simulink model "MyDrivelIne"  (R2018b)
settings: Solver=VariableStepAuto  StartTime=0.0  StopTime=10.0  RelTol=1e-3
libraries: autolibsharedcoupling x3, autolibutils x1, vehdynlibsteering x1, autolibshareddiff x1, autolibsharedtransfixedgear x1
settings Model: Creator=ivory  LastModifiedBy=ivory

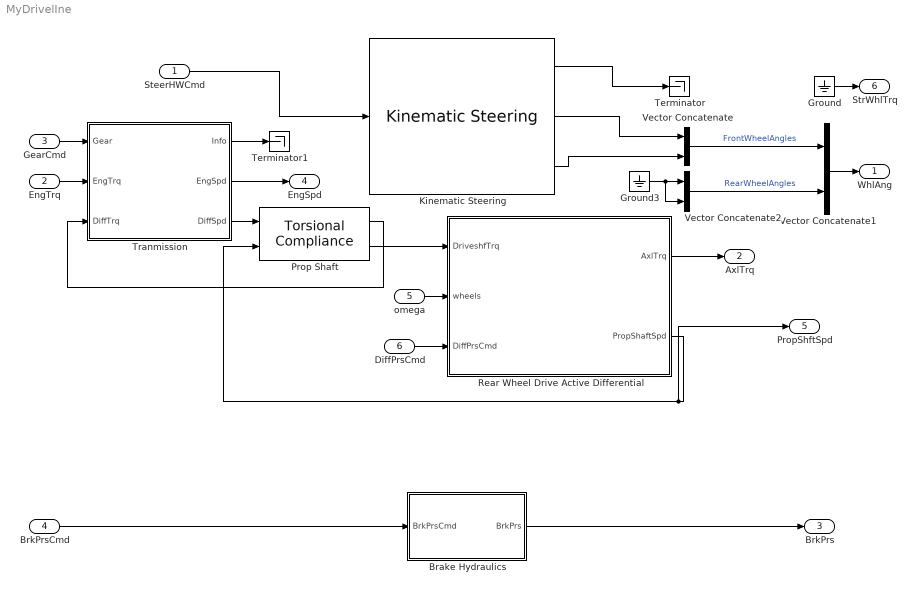
== system MyDrivelIne ==
  SteerHWCmd : Inport
  EngTrq : Inport  Port=2
  GearCmd : Inport  Port=3
  BrkPrsCmd : Inport  Port=4  PortDimensions=4
  omega : Inport  Port=5
  DiffPrsCmd : Inport  Port=6
  Brake Hydraulics : Subsystem
  Ground : Ground
  Ground3 : Ground
  Kinematic Steering : vehdynlibsteering/Kinematic Steering  StrgType=Ackerman  StrgRatioType=Constant  Loc=Front  NrmlFctr=1  TrckWdth=1.922  WhlBase=(1.515+1.504)  Db=0  StrgRng=3*pi  StrgAngBpts="[-6.2832   -5.0265   -3.7699   -2.5133   -1.2566         0    1.2566    2.5133    3.7699    5.0265    6.2832]"  StrgRatioTbl=|  StrgRatio=18  StrgArmLngth=0.1  RckCsLngth=0.5  TieRodLngth=0.248  D=0.2  PnnRadius=0.0057  PnnRadiusTbl="[0.0055    0.0055    0.0056    0.0057    0.0058    0.0057    0.0057    0.0057    0.0056    0.0055    0.0055]"  RodLngth=0.1  ParaArmLngth=0.9  aMode=2
      | [13.5000   13.3750   13.2500   13.1250   13.0000   13.0000   13.0000   13.1250   13.2500   13.3750   13.5000
      | ]
      settings: SourceProductName=Vehicle Dynamics Blockset
  Prop Shaft : autolibsharedcoupling/Torsional Compliance  port_config=Simulink  k=5e3  b=100  theta_o=0  domega_o=0  omega_c=150  blkID=0  aMode=2
      settings: SourceProductName=Powertrain Blockset  SourceProductBaseCode=PW
  Rear Wheel Drive Active Differential : Subsystem
  Terminator : Terminator
  Terminator1 : Terminator
  Tranmission : Subsystem
  Vector Concatenate : Concatenate
  Vector Concatenate1 : Concatenate
  Vector Concatenate2 : Concatenate
  WhlAng : Outport  Unit=rad
  AxlTrq : Outport  Port=2
  BrkPrs : Outport  Port=3  PortDimensions=4
  EngSpd : Outport  Port=4
  PropShftSpd : Outport  Port=5
  StrWhlTrq : Outport  Port=6  Unit=N*m
  wires:
  Ground3/1 -> Vector Concatenate2/2, Vector Concatenate2/1
  Kinematic Steering/1 -> Terminator/1
  Kinematic Steering/3 -> Vector Concatenate/2
  Vector Concatenate1/1 -> WhlAng/1
  Vector Concatenate2/1 -> Vector Concatenate1/2  "RearWheelAngles"
  Vector Concatenate/1 -> Vector Concatenate1/1  "FrontWheelAngles"
  Kinematic Steering/2 -> Vector Concatenate/1
  Ground/1 -> StrWhlTrq/1
  Rear Wheel Drive Active Differential/1(AxlTrq) -> AxlTrq/1
  BrkPrsCmd/1 -> Brake Hydraulics/1(BrkPrsCmd)
  Brake Hydraulics/1(BrkPrs) -> BrkPrs/1
  Tranmission/1(Info) -> Terminator1/1
  Tranmission/2(EngSpd) -> EngSpd/1
  Tranmission/3(DiffSpd) -> Prop Shaft/1
  Prop Shaft/1 -> Tranmission/3(DiffTrq)
  Prop Shaft/2 -> Rear Wheel Drive Active Differential/1(DriveshfTrq)
  omega/1 -> Rear Wheel Drive Active Differential/2(wheels)
  DiffPrsCmd/1 -> Rear Wheel Drive Active Differential/3(DiffPrsCmd)
  Rear Wheel Drive Active Differential/2(PropShaftSpd) -> PropShftSpd/1, Prop Shaft/2
  SteerHWCmd/1 -> Kinematic Steering/1
  EngTrq/1 -> Tranmission/2(EngTrq)
  GearCmd/1 -> Tranmission/1(Gear)

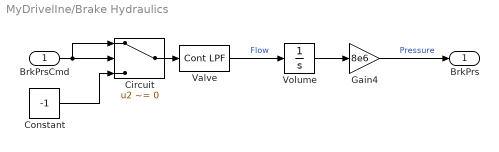
== system MyDrivelIne/Brake Hydraulics ==
  BrkPrsCmd : Inport
  Circuit : Switch  Criteria=u2 ~= 0
  Constant : Constant  Value=-1
  Gain4 : Gain  Gain=8e6
  Valve : autolibutils/Cont LPF  wc=200*2*pi  aMode=2
      settings: SourceProductName=Powertrain Blockset  SourceProductBaseCode=PW
  Volume : Integrator  LimitOutput=on  UpperSaturationLimit=1  LowerSaturationLimit=0  AbsoluteTolerance=1e-3
  BrkPrs : Outport
  wires:
  Volume/1 -> Gain4/1
  Valve/1 -> Volume/1  "Flow"
  BrkPrsCmd/1 -> Circuit/1, Circuit/2
  Gain4/1 -> BrkPrs/1  "Pressure"
  Circuit/1 -> Valve/1
  Constant/1 -> Circuit/3

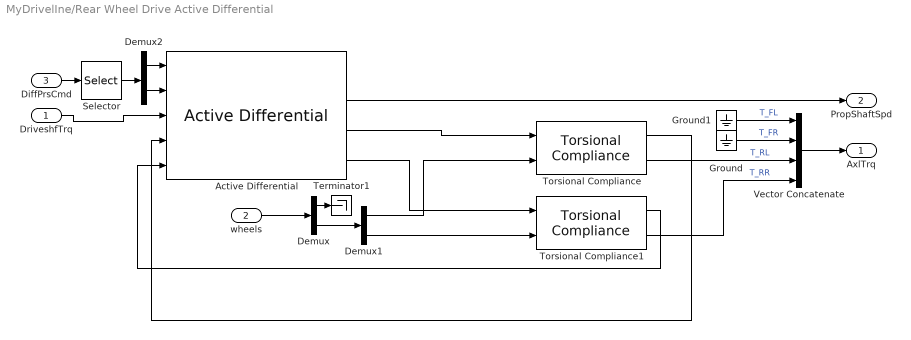
== system MyDrivelIne/Rear Wheel Drive Active Differential ==
  DriveshfTrq : Inport
  wheels : Inport  Port=2
  DiffPrsCmd : Inport  Port=3
  Active Differential : autolibshareddiff/Active Differential  diffType=Spur gears, superposition clutches  Ns1=.875  Ns2=1.125  Jgc=.003  Np1=1.125  Js1=.001  Jc1=.001  Jr1=.002  Np2=1.125  Js2=.001  Jc2=0.001  Jr2=0.002  shaftSwitchMask=To the left of center-line  Ndiff=4  Jd=.1  bd=1e-3  Jw1=.1  bw1=1e-3  Jw2=.1  bw2=1e-3  omegaw1o=0  omegaw2o=0  couplingType=Pre-loaded ideal clutch  Aeff=0.01  Ndisks=4  Reff=.20  Fc=500  muc=[.16 0.13 0.115 0.11 0.105 0.1025 0.10125 .10125]  dw=[0 10 20 40 60 80 100 500]  TdPdw=[-1000, -500, -90, -50, -5, 0, 5, 50, 90, 500, 1000].*ones(11)  pT=[0 1e3 5e3 7e3 1e4 2e4 5e4 1e5 5e5 1e6 5e6]  dwT=[-500 -200, -175, -100, - 50, 0, 50, 100, 175, 200, 500]  tauC=.01  IdealInterpMethod=Linear point-slope  IdealExtrapMethod=Clip  TdwInterpMethod=Linear point-slope  TdwExtrapMethod=Clip  maxAbsSpd=5e3  aMode=2  blkID=0
      settings: SourceProductName=Powertrain Blockset  SourceProductBaseCode=PW
  Demux : Demux  Outputs=[2,2]
  Demux1 : Demux  Outputs=2
  Demux2 : Demux  Outputs=2
  Ground : Ground
  Ground1 : Ground
  Selector : Selector  InputPortWidth=4  IndexOptions=Index vector (dialog)  Indices=[3 4]  OutputSizes=1
  Terminator1 : Terminator
  Torsional Compliance : autolibsharedcoupling/Torsional Compliance  port_config=Simulink  k=5e3  b=50  theta_o=0  domega_o=0  omega_c=150  blkID=0  aMode=2
      settings: SourceProductName=Powertrain Blockset  SourceProductBaseCode=PW
  Torsional Compliance1 : autolibsharedcoupling/Torsional Compliance  port_config=Simulink  k=5e3  b=50  theta_o=0  domega_o=0  omega_c=150  blkID=0  aMode=2
      settings: SourceProductName=Powertrain Blockset  SourceProductBaseCode=PW
  Vector Concatenate : Concatenate  NumInputs=4
  AxlTrq : Outport
  PropShaftSpd : Outport  Port=2
  wires:
  Selector/1 -> Demux2/1
  Ground/1 -> Vector Concatenate/2  "T_FR"
  Ground1/1 -> Vector Concatenate/1  "T_FL"
  Demux1/1 -> Torsional Compliance/2
  Vector Concatenate/1 -> AxlTrq/1
  Demux/1 -> Terminator1/1
  wheels/1 -> Demux/1
  Torsional Compliance1/2 -> Vector Concatenate/4  "T_RR"
  Torsional Compliance/2 -> Vector Concatenate/3  "T_RL"
  Active Differential/2 -> PropShaftSpd/1
  Active Differential/3 -> Torsional Compliance/1
  DiffPrsCmd/1 -> Selector/1
  DriveshfTrq/1 -> Active Differential/3
  Demux2/1 -> Active Differential/1
  Demux2/2 -> Active Differential/2
  Demux/2 -> Demux1/1
  Torsional Compliance/1 -> Active Differential/4
  Torsional Compliance1/1 -> Active Differential/5
  Demux1/2 -> Torsional Compliance1/2
  Active Differential/4 -> Torsional Compliance1/1

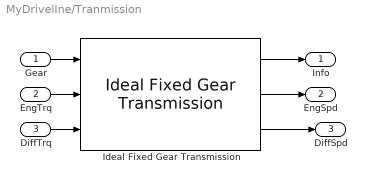
== system MyDrivelIne/Tranmission ==
  Gear : Inport
  EngTrq : Inport  Port=2
  DiffTrq : Inport  Port=3
  Ideal Fixed Gear Transmission : autolibsharedtransfixedgear/Ideal Fixed Gear Transmission  VariantControl=0  TransEffModelPopup=Gear only  gearInterp=Nearest  G=[-1,0,1,2,3,4,5,6,7,8]  Trq_bpts=[25, 50, 75, 100, 150, 200, 250]  omega_bpts=[52.4 78.5 105 131 157 183 209 262 314 419 524]  Temp_bpts=[313 358]  N=[-3.820000000000000,4.560000000000000,4.560000000000000,2.970000000000000,2.080000000000000,1.690000000000000,1.270000000000000,1,0.850000000000000,0.650000000000000]  Jout=[0.128000000000000,0.128000000000000,0.128000000000000,0.100000000000000,0.062000000000000,0.028000000000000,0.010000000000000,0.010000000000000,0.010000000000000,0.010000000000000]  bout=[0.003000000000000,1.000000000000000e-03,0.003000000000000,0.002500000000000,0.002000000000000,1.000000000000000e-03,1.000000000000000e-03,1.000000000000000e-03,1.000000000000000e-03,1.000000000000000e-03]  eta=[0.900000000000000,0.900000000000000,0.900000000000000,0.900000000000000,0.900000000000000,0.950000000000000,0.950000000000000,0.950000000000000,0.950000000000000,0.950000000000000]  eta_tbl=reshape([0.53 0.71 0.77 0.79 0.82 0.82 0.82 0.5 0.7 0.77 0.79 0.82 0.82 0.82 0.54 0.72 0.78 0.81 0.83 0.82 0.82 0.56 0.73 0.79 0.81 0.84 0.82 0.82 0.58 0.74 0.79 0.82 0.84 0.82 0.82 0.57 0.74 0.79 0.82 0.84 0.82 0.82 0.58 0.74 0.79 0.82 0.84 0.82 0.82 0.58 0.74 0.79 0.82 0.84 0.82 0.82 0.57 0.74 0.8 0.82 0.85 0.82 0.82 0.55 0.73 0.78 0.81 0.84 0.82 0.82 0.51 0.71 0.77 0.81 0.84 0.82 0.82 0.53 0.71 0.77 0.79 0.82 0.82 0.82 0.5 0.7 0.77 0.79 0.82 0.82 0.82 0.54 0.72 0.78 0.81 0.83 0.82 0.82 0.56 0.73 0.79 0.81 0.84 0.82 0.82 0.58 0.74 0.79 0.82 0.84 0.82 0.82 0.57 0.74 0.79 0.82 0.84 0.82 0.82 0.58 0.74 0.79 0.82 0.84 0.82 0.82 0.58 0.74 0.79 0.82 0.84 0.82 0.82 0.57 0.74 0.8 0.82 0.85 0.82 0.82 0.55 0.73 0.78 0.81 0.84 0.82 0.82 0.51 0.71 0.77 0.81 0.84 0.82 0.82 0.53 0.71 0.77 0.79 0.82 0.82 0.82 0.5 0.7 0.77 0.79 0.82 0.82 0.82 0.54 0.72 0.78 0.81 0.83 0.82 0.82 0.56 0.73 0.79 0.81 0.84 0.82 0.82 0.58 0.74 0.79 0.82 0.84 0.82 0.82 0.57 0.74 0.79 0.82 0.84 0.82 0.82 0.58 0.74 0.79 0.82 0.84 0.82 0.82 0.58 0.74 0.79 0.82 0.84 0.82 0.82 0.57 0.74 0.8 0.82 0.85 0.82 0.82 0.55 0.73 0.78 0.81 0.84 0.82 0.82 0.51 0.71 0.77 0.81 0.84 0.82 0.82 0.7 0.79 0.82 0.83 0.84 0.84 0.84 0.63 0.76 0.8 0.82 0.83 0.84 0.84 0.58 0.74 0.79 0.81 0.83 0.84 0.84 0.58 0.74 0.79 0.81 0.83 0.84 0.84 0.58 0.74 0.79 0.81 0.84 0.84 0.84 0.57 0.73 0.78 0.81 0.84 0.85 0.84 0.57 0.73 0.79 0.81 0.84 0.85 0.84 0.56 0.73 0.78 0.81 0.83 0.85 0.84 0.55 0.73 0.78 0.81 0.84 0.85 0.84 0.52 0.71 0.77 0.8 0.83 0.85 0.84 0.48 0.69 0.76 0.79 0.83 0.84 0.84 0.64 0.76 0.8 0.81 0.83 0.84 0.84 0.56 0.73 0.78 0.8 0.83 0.84 0.84 0.54 0.71 0.77 0.8 0.82 0.84 0.84 0.53 0.71 0.77 0.8 0.83 0.84 0.84 0.51 0.71 0.77 0.8 0.83 0.84 0.85 0.52 0.7 0.77 0.8 0.83 0.84 0.85 0.51 0.71 0.76 0.79 0.83 0.84 0.85 0.5 0.69 0.76 0.79 0.82 0.84 0.85 0.45 0.68 0.75 0.78 0.82 0.84 0.85 0.43 0.67 0.74 0.78 0.81 0.83 0.84 0.38 0.63 0.71 0.75 0.8 0.82 0.83 0.65 0.79 0.84 0.85 0.88 0.89 0.89 0.56 0.75 0.81 0.83 0.86 0.88 0.89 0.52 0.72 0.79 0.83 0.86 0.88 0.88 0.51 0.72 0.79 0.83 0.86 0.88 0.89 0.49 0.71 0.78 0.82 0.86 0.88 0.89 0.47 0.7 0.78 0.82 0.86 0.87 0.88 0.45 0.69 0.77 0.81 0.85 0.87 0.88 0.4 0.67 0.75 0.8 0.84 0.86 0.88 0.3 0.64 0.73 0.78 0.83 0.86 0.87 0.17 0.55 0.67 0.73 0.8 0.83 0.85 0.089 0.45 0.61 0.69 0.77 0.81 0.83 0.61 0.75 0.82 0.84 0.87 0.87 0.88 0.54 0.73 0.8 0.82 0.86 0.87 0.88 0.51 0.71 0.79 0.82 0.86 0.87 0.88 0.52 0.72 0.79 0.82 0.86 0.87 0.89 0.52 0.72 0.8 0.83 0.86 0.88 0.89 0.53 0.72 0.79 0.82 0.86 0.87 0.89 0.5 0.7 0.78 0.82 0.86 0.88 0.88 0.46 0.69 0.77 0.81 0.85 0.87 0.88 0.4 0.67 0.75 0.8 0.83 0.86 0.88 0.33 0.64 0.73 0.78 0.83 0.85 0.87 0.33 0.64 0.73 0.78 0.83 0.85 0.87 0.78 0.85 0.87 0.88 0.89 0.89 0.89 0.73 0.83 0.86 0.88 0.89 0.89 0.89 0.72 0.83 0.86 0.88 0.89 0.89 0.89 0.72 0.83 0.87 0.89 0.9 0.89 0.89 0.72 0.83 0.87 0.88 0.9 0.89 0.89 0.71 0.83 0.87 0.88 0.9 0.89 0.89 0.71 0.83 0.86 0.88 0.9 0.89 0.89 0.7 0.82 0.86 0.88 0.9 0.89 0.89 0.69 0.82 0.86 0.88 0.9 0.89 0.89 0.67 0.81 0.86 0.88 0.9 0.89 0.89 0.63 0.79 0.85 0.87 0.89 0.89 0.89 0.78 0.85 0.87 0.88 0.89 0.89 0.89 0.73 0.83 0.86 0.88 0.89 0.89 0.89 0.72 0.83 0.86 0.88 0.89 0.89 0.89 0.72 0.83 0.87 0.89 0.9 0.89 0.89 0.72 0.83 0.87 0.88 0.9 0.89 0.89 0.71 0.83 0.87 0.88 0.9 0.89 0.89 0.71 0.83 0.86 0.88 0.9 0.89 0.89 0.7 0.82 0.86 0.88 0.9 0.89 0.89 0.69 0.82 0.86 0.88 0.9 0.89 0.89 0.67 0.81 0.86 0.88 0.9 0.89 0.89 0.63 0.79 0.85 0.87 0.89 0.89 0.89 0.78 0.85 0.87 0.88 0.89 0.89 0.89 0.73 0.83 0.86 0.88 0.89 0.89 0.89 0.72 0.83 0.86 0.88 0.89 0.89 0.89 0.72 0.83 0.87 0.89 0.9 0.89 0.89 0.72 0.83 0.87 0.88 0.9 0.89 0.89 0.71 0.83 0.87 0.88 0.9 0.89 0.89 0.71 0.83 0.86 0.88 0.9 0.89 0.89 0.7 0.82 0.86 0.88 0.9 0.89 0.89 0.69 0.82 0.86 0.88 0.9 0.89 0.89 0.67 0.81 0.86 0.88 0.9 0.89 0.89 0.63 0.79 0.85 0.87 0.89 0.89 0.89 0.82 0.87 0.88 0.89 0.89 0.89 0.89 0.81 0.87 0.89 0.89 0.9 0.9 0.89 0.76 0.85 0.87 0.89 0.9 0.89 0.89 0.72 0.83 0.86 0.88 0.89 0.89 0.89 0.72 0.83 0.86 0.88 0.89 0.9 0.89 0.71 0.82 0.86 0.88 0.89 0.9 ...(+1314 chars))  omega_o=0  tau_s=0.020000000000000  maxAbsSpd=5e3  aMode=2
      settings: SourceProductName=Powertrain Blockset  SourceProductBaseCode=PW
  Info : Outport
  EngSpd : Outport  Port=2
  DiffSpd : Outport  Port=3
  wires:
  Gear/1 -> Ideal Fixed Gear Transmission/1
  EngTrq/1 -> Ideal Fixed Gear Transmission/2
  DiffTrq/1 -> Ideal Fixed Gear Transmission/3
  Ideal Fixed Gear Transmission/1 -> Info/1
  Ideal Fixed Gear Transmission/2 -> EngSpd/1
  Ideal Fixed Gear Transmission/3 -> DiffSpd/1
